simulink model "chap8_1sim"  (Simulink 7.7)
settings: Solver=ode45  StartTime=0.0  StopTime=20  RelTol=1e-3
settings Model: Creator=guozhu  LastModifiedBy=ljk
settings DataIOCC: SignalLoggingName=sigsOut
settings DebuggingCC: SaveWithParameterizedLinksMsg=none  SignalResolutionControl=TryResolveAllWithWarning  SolverPrmCheckMsg=none  MultiTaskDSMMsg=warning  MultiTaskCondExecSysMsg=none  StrictBusMsg=Warning
settings HardwareCC: TargetUnknown=on
settings RTWCC: IncludeERTFirstTime=on

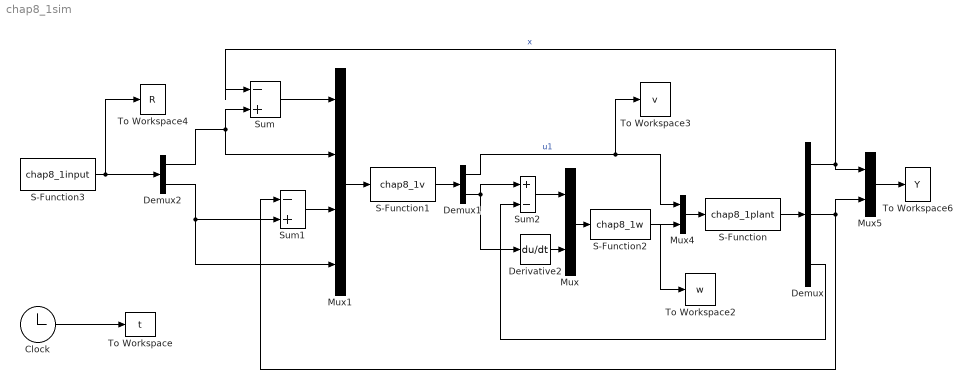
== system chap8_1sim ==
  Clock : Clock
  Demux : Demux  Outputs=3
  Demux1 : Demux  Outputs=2
  Demux2 : Demux  Outputs=2
  Derivative2 : Derivative
  Mux : Mux  Inputs=2
  Mux1 : Mux
  Mux4 : Mux  Inputs=2
  Mux5 : Mux  Inputs=2
  S-Function : S-Function  FunctionName=chap8_1plant  EnableBusSupport=off
  S-Function1 : S-Function  FunctionName=chap8_1v  EnableBusSupport=off
  S-Function2 : S-Function  FunctionName=chap8_1w  EnableBusSupport=off
  S-Function3 : S-Function  FunctionName=chap8_1input  EnableBusSupport=off
  Sum : Sum  Inputs=|-+  SaturateOnIntegerOverflow=on
  Sum1 : Sum  Inputs=|-+  SaturateOnIntegerOverflow=on
  Sum2 : Sum  Inputs=|+-  SaturateOnIntegerOverflow=on
  To Workspace : ToWorkspace  VariableName=t  SampleTime=-1  SaveFormat=Array
  To Workspace2 : ToWorkspace  VariableName=w  SampleTime=-1  SaveFormat=Array
  To Workspace3 : ToWorkspace  VariableName=v  SampleTime=-1  SaveFormat=Array
  To Workspace4 : ToWorkspace  VariableName=R  SampleTime=-1  SaveFormat=Array
  To Workspace6 : ToWorkspace  VariableName=Y  SampleTime=-1  SaveFormat=Array
  wires:
  S-Function/1 -> Demux/1
  Demux/1 -> Mux5/1, Sum/1  "x"
  Mux1/1 -> S-Function1/1
  Demux/2 -> Mux5/2, Sum1/1
  Demux2/1 -> Sum/2, Mux1/2
  Sum1/1 -> Mux1/3
  Demux2/2 -> Sum1/2, Mux1/4
  S-Function1/1 -> Demux1/1
  Sum/1 -> Mux1/1
  Demux1/2 -> Derivative2/1, Sum2/1
  Mux/1 -> S-Function2/1
  S-Function2/1 -> To Workspace2/1, Mux4/2
  Demux1/1 -> Mux4/1, To Workspace3/1  "u1"
  Mux4/1 -> S-Function/1
  Derivative2/1 -> Mux/2
  Clock/1 -> To Workspace/1
  Demux/3 -> Sum2/2
  Sum2/1 -> Mux/1
  Mux5/1 -> To Workspace6/1
  S-Function3/1 -> Demux2/1, To Workspace4/1
